simulink model "test2"  (R2016a)
settings: Solver=ode4  StartTime=0.0  StopTime=inf  RelTol=1e-3
model workspace (MAT data in the model file):
  RDTCommand.header = 4660
  RDTCommand.command = 1
  RDTCommand.count = 0
  addr : java.net.Inet4Address (value not decoded)
  atiData.RDTPORT = 49152
  atiData.LOCALPORT = 9091
  atiData.NetBoxIP = '192.168.1.1'
  atiData.calmat = [1 1 1 25 25 35 250 250 250]
  atiData.packetLength = 36
  atiData.headerMessage = 4660
  atiData.packetCount = 0
  atiData.packet = []
  dataGramPacketRDT = [18 52 0 1 0 0 0 0]
  dpath = {'D:\ATI\Matlab\ATINetFT.jar'}
libraries: slrtlib x7, xpcmeasurementcomputinglib x5, xpcconteclib x2
settings Model: SimulationMode=external  Creator=Biorobotics  LastModifiedBy=Biorobotics
settings SolverCC: EnableConcurrentExecution=on
settings DataIOCC: SaveFormat=StructureWithTime
settings OptimizationCC: BlockReduction=off  OptimizeBlockIOStorage=off  BufferReuse=off  GlobalBufferReuse=off  ExpressionFolding=off  LocalBlockOutputs=off
settings HardwareCC: ProdBitPerPointer=32  ProdLargestAtomicFloat=None  ProdWordSize=32  ProdLongLongMode=on  ProdHWDeviceType=Generic->32-bit x86 compatible
settings RTWCC: SystemTargetFile=slrt.tlc  TemplateMakefile=slrt_default_tmf  Description=Simulink Real-Time  RTWCompilerOptimization=on

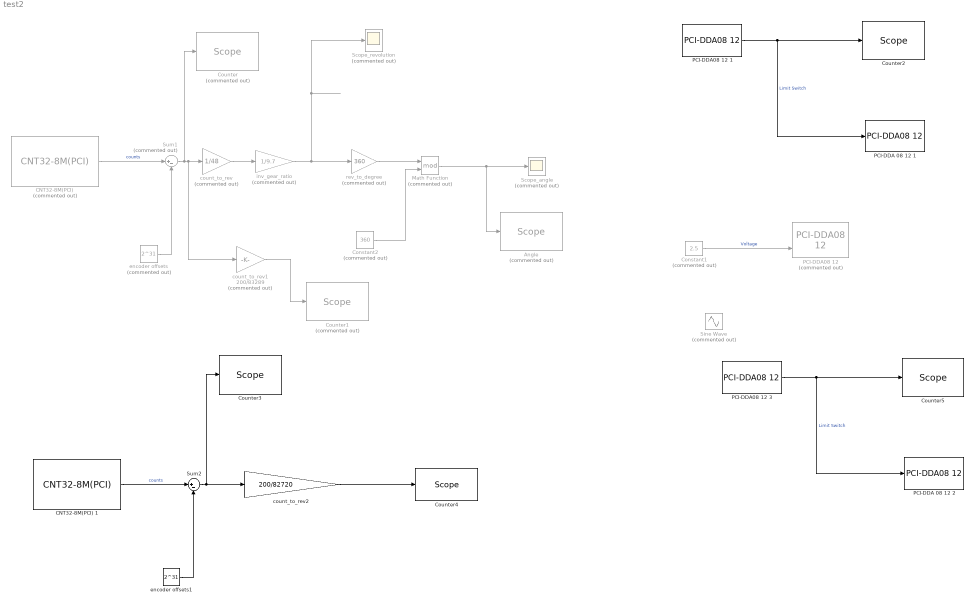
== system test2 ==
  Angle : slrtlib/Displays and Logging/Scope   Commented=on  scopeno=4  scopetype=Target  autostart=on  viewmode=Numerical  formatstr='%15.6f'  grid=on  ylimits=[0,0]  nosamples=1000  noprepostsamples=0  interleave=1  triggermode=FreeRun  triggersignal=1  trigsignalfromport=off  triggerlevel=0.0  triggerslope=Either  triggerscope=1  triggersample=0  filename=data.dat  mode=Lazy  writesize=512  autorestart=off  dynamicfilemode=off  maxwritefilesize=512*1024^2
  "CNT32-8M(PCI) " : xpcconteclib/Incremental Encoder/CNT32-8M(PCI)   Commented=on  Channel=1  OperationMode=2-phase Input Synchronous Clear Multiply by 4  DigitalFilter=No filtering  PulseInput=TTL level input  Direction=Up in the clockwise direction/Down in the counterclockwise direction  InitialValue=2^31  LoadInitialValue=on  SampleTime=0.0001  PciSlot=[4 5]  StartMethod=Model Start  StopMethod=Model Terminate  ZeroClearRising=off  ZeroClearFalling=off  ZeroClearMatch0=off  ZeroClearMatch1=off  PresetRising=off  PresetFalling=off  PresetMatch0=off  PresetMatch1=off  PresetValue=0  Match0Value=0  Match1Value=0  OutputSignalMatch0=off  OutputSignalMatch1=off  OutputSignalAbnormal=off  OutputSignalDigitalFilter=off  OutputSignalAlarm=off  OneShotDuration=10 microseconds  IndexEnable=Disable  IndexLogic=Positive (Active High)  EnableDigitalInput=off  EnableDigitalOutput=off  DigitalOutputInitialValue=None  DigitalOutputFinalValue=None
  CNT32-8M(PCI) 1 : xpcconteclib/Incremental Encoder/CNT32-8M(PCI)   Channel=4  OperationMode=2-phase Input Synchronous Clear Multiply by 4  DigitalFilter=No filtering  PulseInput=TTL level input  Direction=Up in the clockwise direction/Down in the counterclockwise direction  InitialValue=2^31  LoadInitialValue=on  SampleTime=0.0001  PciSlot=[4 5]  StartMethod=Model Start  StopMethod=Model Terminate  ZeroClearRising=off  ZeroClearFalling=off  ZeroClearMatch0=off  ZeroClearMatch1=off  PresetRising=off  PresetFalling=off  PresetMatch0=off  PresetMatch1=off  PresetValue=0  Match0Value=0  Match1Value=0  OutputSignalMatch0=off  OutputSignalMatch1=off  OutputSignalAbnormal=off  OutputSignalDigitalFilter=off  OutputSignalAlarm=off  OneShotDuration=10 microseconds  IndexEnable=Disable  IndexLogic=Positive (Active High)  EnableDigitalInput=off  EnableDigitalOutput=off  DigitalOutputInitialValue=None  DigitalOutputFinalValue=None
  Constant1 : Constant  Commented=on  Value=2.5
  Constant2 : Constant  Commented=on  Value=360
  Counter : slrtlib/Displays and Logging/Scope   Commented=on  scopeno=3  scopetype=Target  autostart=on  viewmode=Numerical  formatstr='%15.6f'  grid=on  ylimits=[0,0]  nosamples=10000  noprepostsamples=0  interleave=1  triggermode=FreeRun  triggersignal=1  trigsignalfromport=off  triggerlevel=0.0  triggerslope=Either  triggerscope=1  triggersample=0  filename=data.dat  mode=Lazy  writesize=512  autorestart=off  dynamicfilemode=off  maxwritefilesize=512*1024^2
  Counter1 : slrtlib/Displays and Logging/Scope   Commented=on  scopeno=1  scopetype=Target  autostart=on  viewmode=Numerical  formatstr='%15.6f'  grid=on  ylimits=[0,0]  nosamples=10000  noprepostsamples=0  interleave=1  triggermode=FreeRun  triggersignal=1  trigsignalfromport=off  triggerlevel=0.0  triggerslope=Either  triggerscope=1  triggersample=0  filename=data.dat  mode=Lazy  writesize=512  autorestart=off  dynamicfilemode=off  maxwritefilesize=512*1024^2
  Counter2 : slrtlib/Displays and Logging/Scope   scopeno=2  scopetype=Target  autostart=on  viewmode=Numerical  formatstr='%15.6f'  grid=on  ylimits=[0,0]  nosamples=1000  noprepostsamples=0  interleave=1  triggermode=FreeRun  triggersignal=1  trigsignalfromport=off  triggerlevel=0.0  triggerslope=Either  triggerscope=1  triggersample=0  filename=data.dat  mode=Lazy  writesize=512  autorestart=off  dynamicfilemode=off  maxwritefilesize=512*1024^2
  Counter3 : slrtlib/Displays and Logging/Scope   scopeno=4  scopetype=Target  autostart=on  viewmode=Numerical  formatstr='%15.6f'  grid=on  ylimits=[0,0]  nosamples=3  noprepostsamples=0  interleave=1  triggermode=FreeRun  triggersignal=1  trigsignalfromport=off  triggerlevel=0.0  triggerslope=Either  triggerscope=1  triggersample=0  filename=data.dat  mode=Lazy  writesize=512  autorestart=off  dynamicfilemode=off  maxwritefilesize=512*1024^2
  Counter4 : slrtlib/Displays and Logging/Scope   scopeno=5  scopetype=Target  autostart=on  viewmode=Graphical rolling  formatstr='%15.6f'  grid=on  ylimits=[0,0]  nosamples=500  noprepostsamples=0  interleave=1  triggermode=FreeRun  triggersignal=1  trigsignalfromport=off  triggerlevel=0.0  triggerslope=Either  triggerscope=1  triggersample=0  filename=data.dat  mode=Lazy  writesize=512  autorestart=off  dynamicfilemode=off  maxwritefilesize=512*1024^2
  Counter5 : slrtlib/Displays and Logging/Scope   scopeno=6  scopetype=Target  autostart=on  viewmode=Numerical  formatstr='%15.6f'  grid=on  ylimits=[0,0]  nosamples=1000  noprepostsamples=0  interleave=1  triggermode=FreeRun  triggersignal=1  trigsignalfromport=off  triggerlevel=0.0  triggerslope=Either  triggerscope=1  triggersample=0  filename=data.dat  mode=Lazy  writesize=512  autorestart=off  dynamicfilemode=off  maxwritefilesize=512*1024^2
  Math Function : Math  Commented=on  Operator=mod  SaturateOnIntegerOverflow=on
  PCI-DDA 08 12 1 : xpcmeasurementcomputinglib/Digital Output/PCI-DDA08 12   channel=1  port=A  reset=[1]  initValue=[0]  chip=1  sampletime=0.001  slot=-1
  PCI-DDA 08 12 2 : xpcmeasurementcomputinglib/Digital Output/PCI-DDA08 12   channel=3  port=A  reset=[1]  initValue=[0]  chip=1  sampletime=0.001  slot=-1
  "PCI-DDA08 12 " : xpcmeasurementcomputinglib/D//A/PCI-DDA08 12   Commented=on  channel=[1 2]  range=[-10 -10]  reset=[1]  initValue=[0]  sampletime=0.001  pci_dev=-1
  PCI-DDA08 12 1 : xpcmeasurementcomputinglib/Digital Input/PCI-DDA08 12   channel=6  port=A  chip=2  sampletime=0.001  slot=-1
  PCI-DDA08 12 3 : xpcmeasurementcomputinglib/Digital Input/PCI-DDA08 12   channel=6  port=B  chip=2  sampletime=0.001  slot=-1
  Scope_angle : Scope  Commented=on
  Scope_revolution : Scope  Commented=on
  Sine Wave : Sin  Commented=on  SineType=Sample based  Amplitude=3  Frequency=0.5  Samples=10000  SampleTime=0.001
  Sum1 : Sum  Commented=on  Inputs=|+-
  Sum2 : Sum  Inputs=|+-
  count_to_rev : Gain  Commented=on  Gain=1/48
  count_to_rev1 : Gain  Commented=on  Gain=200/83289
  count_to_rev2 : Gain  Gain=200/82720
  encoder offsets : Constant  Commented=on  Value=2^31
  encoder offsets1 : Constant  Value=2^31
  inv_gear_ratio : Gain  Commented=on  Gain=1/9.7
  rev_to_degree : Gain  Commented=on  Gain=360
  wires:
  encoder offsets/1 -> Sum1/2
  "CNT32-8M(PCI) "/1 -> Sum1/1  "counts"
  inv_gear_ratio/1 -> Scope_revolution/1, rev_to_degree/1
  Sum1/1 -> Counter/1, count_to_rev1/1, count_to_rev/1
  rev_to_degree/1 -> Math Function/1
  Math Function/1 -> Angle/1, Scope_angle/1
  Constant2/1 -> Math Function/2
  count_to_rev/1 -> inv_gear_ratio/1
  count_to_rev1/1 -> Counter1/1
  PCI-DDA08 12 1/1 -> PCI-DDA 08 12 1/1, Counter2/1  "Limit Switch"
  encoder offsets1/1 -> Sum2/2
  CNT32-8M(PCI) 1/1 -> Sum2/1  "counts"
  Sum2/1 -> Counter3/1, count_to_rev2/1
  count_to_rev2/1 -> Counter4/1
  PCI-DDA08 12 3/1 -> PCI-DDA 08 12 2/1, Counter5/1  "Limit Switch"
  Constant1/1 -> "PCI-DDA08 12 "/2  "Voltage"
